simulink model "MPC_MMC_qudratic_FPGA_y_limit"  (R2022a)
settings: Solver=ode3  StartTime=0.0  StopTime=3  FixedStep=0.000050  RelTol=1e-3  EnableMultiTasking=on
settings Model: Creator=cary  LastModifiedBy=adshetgaonkar
settings SolverCC: AlgebraicLoopSolver=TrustRegion
settings DataIOCC: LimitDataPoints=on  SaveFormat=Array  SignalLoggingSaveFormat=ModelDataLogs  ReturnWorkspaceOutputs=off
settings OptimizationCC: ExpressionDepthLimit=2147483647  LifeSpan=1  EfficientTunableParamExpr=on
settings DebuggingCC: UnderspecifiedInitializationDetection=Classic  MergeDetectMultiDrivingBlocksExec=none  SolverPrmCheckMsg=warning  FcnCallInpInsideContextMsg=warning  UnconnectedInputMsg=warning  UnconnectedOutputMsg=warning  UnconnectedLineMsg=warning  StateNameClashWarn=warning  SFUnexpectedBacktrackingDiag=warning  SFNoUnconditionalDefaultTransitionDiag=warning  SFExecutionAtInitializationDiag=none  SFMachineParentedDataDiag=warning  ArithmeticOperatorsInVariantConditions=warning
settings HardwareCC: ProdBitPerPointer=32  ProdBitPerSizeT=32  ProdBitPerPtrDiffT=32  ProdLargestAtomicFloat=None  ProdIntDivRoundTo=Undefined  ProdEndianess=Unspecified  ProdWordSize=32  ProdHWDeviceType=32-bit Generic
settings ModelReferenceCC: PropagateSignalLabelsOutOfModel=off
settings SFSimCC: SimUseLocalCustomCode=off  MATLABDynamicMemAlloc=off  CustomCodeUndefinedFunction=UseInterfaceOnly
settings RTWCC: SystemTargetFile=ert.tlc  TemplateMakefile=ert_default_tmf  RTWUseLocalCustomCode=off
settings CodeAppCC: IgnoreCustomStorageClasses=off  CustomSymbolStrType=$N$R$M  StateflowObjectComments=on  InternalIdentifier=Classic
settings ERTTargetCC: MultiwordLength=2048  GenerateSampleERTMain=on  IncludeMdlTerminateFcn=off  SupportComplex=off  SupportContinuousTime=on  ERTCustomFileTemplate=example_file_process.tlc  ConvertIfToSwitch=off  SuppressUnreachableDefaultCases=off
settings ConfigComp: CovMetricSettings=dw  CovSaveCumulativeToWorkspaceVar=on  CovSaveSingleToWorkspaceVar=on  CovExternalEMLEnable=off

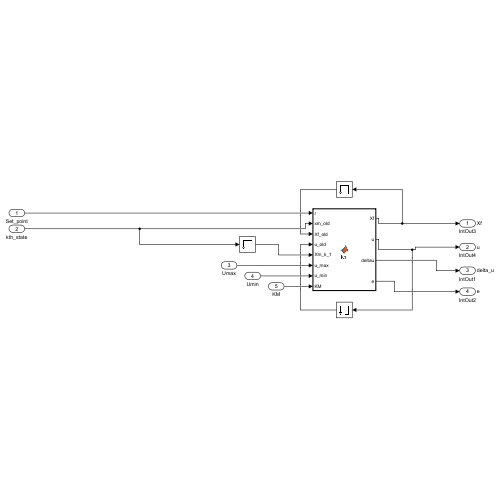
[thumbnail: Simulink's stored preview of the top-level diagram]
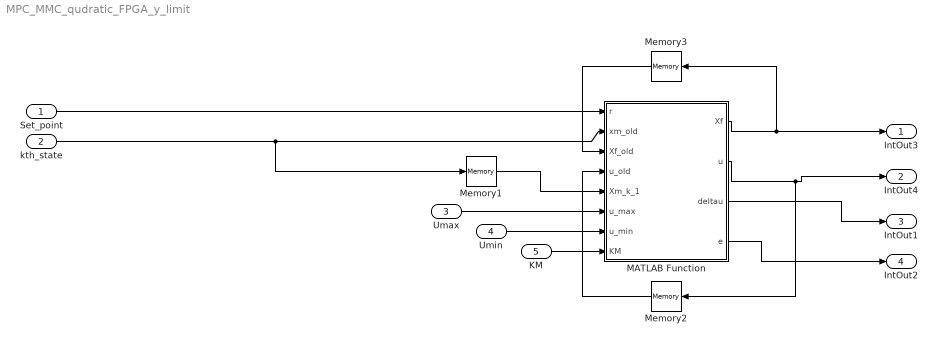
== system MPC_MMC_qudratic_FPGA_y_limit ==
  Set_point : Inport  PortDimensions=5
  kth_state : Inport  Port=2  PortDimensions=5
  Umax : Inport  Port=3  PortDimensions=5
  Umin : Inport  Port=4  PortDimensions=5
  KM : Inport  Port=5  PortDimensions=5
  MATLAB Function : MATLAB Function  TreatAsAtomicUnit=on
  Memory1 : Memory
  Memory2 : Memory
  Memory3 : Memory
  IntOut3 : Outport  SignalName=Xf
  IntOut4 : Outport  Port=2  SignalName=u
  IntOut1 : Outport  Port=3  SignalName=delta_u
  IntOut2 : Outport  Port=4  SignalName=e
  wires:
  Set_point/1 -> MATLAB Function/1(r)
  MATLAB Function/1(Xf) -> Memory3/1, IntOut3/1
  kth_state/1 -> MATLAB Function/2(xm_old), Memory1/1
  MATLAB Function/3(deltau) -> IntOut1/1
  Memory1/1 -> MATLAB Function/5(Xm_k_1)
  Memory3/1 -> MATLAB Function/3(Xf_old)
  Memory2/1 -> MATLAB Function/4(u_old)
  MATLAB Function/2(u) -> IntOut4/1, Memory2/1
  Umax/1 -> MATLAB Function/6(u_max)
  Umin/1 -> MATLAB Function/7(u_min)
  KM/1 -> MATLAB Function/8(KM)
  MATLAB Function/4(e) -> IntOut2/1

== matlab function MPC_MMC_qudratic_FPGA_y_limit/MATLAB Function ==
  data: r input; Xf output; xm_old input; u output; Xf_old input; u_old input; Xm_k_1 input; deltau output; u_max input; u_min input; KM input; e output
function [Xf,u,deltau,e] = fcn(r,xm_old,Xf_old,u_old,Xm_k_1,u_max,u_min,KM)
D = []; 
D= coder.load('initial_qudratic_paper_FPGAv2.mat'); 

xm=D.Ap_ac*xm_old+D.Bp_ac*(u_old+D.up);
y_model=D.Cp_ac*xm;
e = (y_model - xm_old); 

%gamma=[(u_max - u_old);(-u_min + u_old); D.deltau_max; -D.deltau_min;D.yMax - D.C_F*(D.Xf+Xf_old); -D.yMin + D.C_F*(D.Xf+Xf_old)]
gamma=[(u_max - u_old);(-u_min + u_old); D.deltau_max; -D.deltau_min];
eta = QPhild(D.Omega,D.Psi*(D.Xf+Xf_old),D.M,gamma,KM);
%eta= -(D.Omega\D.Psi)*(D.Xf+Xf_old);
deltau= D.Lzerot*eta;
u=D.up+u_old+deltau;
y = xm_old;
y_delta_k=y-Xm_k_1;
Xf=[y_delta_k;y-r];
end
